simulink model "TCR_Simulation"  (R2024a)
settings: Solver=VariableStepAuto  StartTime=0.0  StopTime=0.1  MaxStep=1e-5  RelTol=1e-3
values from neighbouring files (symbols this model uses):
  a = angles(i)    [TCR_Simulation_Matlab.m]    (also in plot_TCR.m)
libraries: spsCurrentMeasurementLib x2, spsSeriesRLCBranchLib x2, spsThyristorLib x2, spsACVoltageSourceLib x1, spsVoltageMeasurementLib x1, sps_lib x1
settings Model: Creator=E370_  LastModifiedBy=E370_

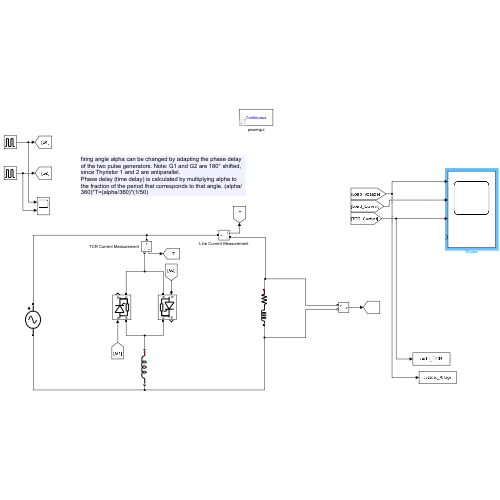
[thumbnail: Simulink's stored preview of the top-level diagram]
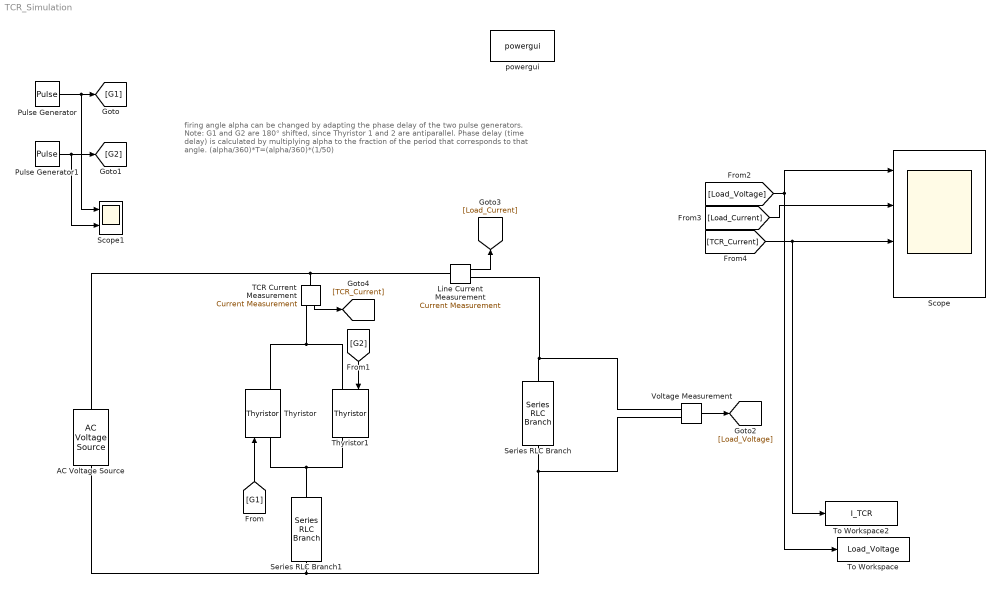
== system TCR_Simulation ==
  note: firing angle alpha can be changed by adapting the phase delay
      | of the two pulse generators. Note: G1 and G2 are 180° shifted, since Thyristor 1 and 2 are antiparallel.
      | Phase delay (time delay) is calculated by multiplying alpha to the fraction of the period that corresponds to that angle. (alpha/360)*T=(alpha/360)*(1/50)
  AC Voltage Source : spsACVoltageSourceLib/AC Voltage Source  Amplitude=100*sqrt(2)  Phase=0  Frequency=50  SampleTime=0  Measurements=None  BusType=swing  Pref=10e3  Qref=0  Qmin=-inf  Qmax=+inf
  Line Current Measurement : spsCurrentMeasurementLib/Current Measurement  PhasorSimulation=off  OutputType=Complex  PSBequivalent=0
  Pulse Generator : DiscretePulseGenerator  PulseType=Time based  Period=1/50  PulseWidth=5  PhaseDelay=(1/50)*((180+a)/360)
  Pulse Generator1 : DiscretePulseGenerator  PulseType=Time based  Period=1/50  PulseWidth=5  PhaseDelay=(1/50)*(a/360)
  Scope : Scope  NumInputPorts=4
  Scope1 : Scope  NumInputPorts=2
  Series RLC Branch : spsSeriesRLCBranchLib/Series RLC Branch  LConnTagsString=__new0  RConnTagsString=__new0  BranchType=RL  Resistance=3.8  Inductance=11e-3  SetiL0=off  InitialCurrent=0  Capacitance=1e-6  Setx0=off  InitialVoltage=0  Measurements=None
  Series RLC Branch1 : spsSeriesRLCBranchLib/Series RLC Branch  LConnTagsString=__new0  RConnTagsString=__new0  BranchType=L  Resistance=3.8  Inductance=5e-3  SetiL0=off  InitialCurrent=0  Capacitance=1e-6  Setx0=off  InitialVoltage=0  Measurements=None
  TCR Current Measurement : spsCurrentMeasurementLib/Current Measurement  PhasorSimulation=off  OutputType=Complex  PSBequivalent=0
  Thyristor : spsThyristorLib/Thyristor  Ron=0.001  Lon=0  Vf=0.8  IC=0  Rs=500  Cs=250e-9  Measurements=on
  Thyristor1 : spsThyristorLib/Thyristor  Ron=0.001  Lon=0  Vf=0.8  IC=0  Rs=500  Cs=250e-9  Measurements=on
  To Workspace : ToWorkspace  VariableName=Load_Voltage  SaveFormat=Timeseries  SampleTime=-1
  To Workspace2 : ToWorkspace  VariableName=I_TCR  SaveFormat=Timeseries  SampleTime=-1
  Voltage Measurement : spsVoltageMeasurementLib/Voltage Measurement  PhasorSimulation=off  OutputType=Complex  PSBequivalent=0
  powergui : sps_lib/powergui  Priority=1  SimulationMode=Continuous  SampleTime=50e-6  frequency=60  Iterations=50  frequencyindice=50  Pbase=100e6  ErrMax=1e-4  UnitsV=kV  UnitsW=MW  buscounter=0  FunctionMessages=off  echomessages=off  EnableUseOfTLC=off  CurrentSourceSwitches=off  DisableSnubberDevices=off  DisableRonSwitches=off  DisableVfSwitches=off  DisplayEquations=off  AutomaticDiscreteSolvers=off  SolverType=Tustin/Backward Euler (TBE)  Interpol=off  ExternalGateDelay=off  methode=off  Ts=100  x0status=blocks  SPID=on  SwTol=0  HookPort=off  NonlinearTolerance=1e-4  nMaxIteration=100  ContinueOnMaxIteration=off  RestoreLinks=warning  ResistiveCurrentMeasurement=off  Frange=[0:2:500]  Ylog=off  Xlog=on  ShowGrid=off  save=off  variable=ZData  structure=0  ZoomFFT=off  StartTime=0.0  cycles=1  DisplayStyle=1  fundamental=60  FreqAxis=off  MaxFrequency=1000  frequencyindicesteady=1  RmsSteady=1  display=off
  wires:
  Pulse Generator/1 -> Scope1/1, [G1]
  Pulse Generator1/1 -> Scope1/2, [G2]
  [G1] -> Thyristor/1
  [G2] -> Thyristor1/1
  Voltage Measurement/1 -> [Load_Voltage]
  [Load_Voltage] -> To Workspace/1, Scope/1
  Line Current Measurement/1 -> [Load_Current]
  [Load_Current] -> Scope/2
  TCR Current Measurement/1 -> [TCR_Current]
  [TCR_Current] -> To Workspace2/1, Scope/3
  connections:
  Thyristor/LConn1 -- Thyristor1/RConn1 -- Series RLC Branch1/LConn1
  AC Voltage Source/LConn1 -- Voltage Measurement/LConn2 -- Series RLC Branch/RConn1 -- Series RLC Branch1/RConn1
  Series RLC Branch/LConn1 -- Line Current Measurement/RConn1 -- Voltage Measurement/LConn1
  Thyristor/RConn1 -- TCR Current Measurement/RConn1 -- Thyristor1/LConn1
  Line Current Measurement/LConn1 -- TCR Current Measurement/LConn1 -- AC Voltage Source/RConn1
